simulink model "DSM6"  (R2020a)
settings: Solver=VariableStepAuto  StartTime=0.0  StopTime=0.3  RelTol=1e-3
settings Model: Creator=86188  LastModifiedBy=bzhan
settings DataIOCC: ReturnWorkspaceOutputs=off
settings DebuggingCC: ArithmeticOperatorsInVariantConditions=warning
settings SFSimCC: SimUseLocalCustomCode=off  CustomCodeUndefinedFunction=UseInterfaceOnly
settings RTWCC: RTWUseLocalCustomCode=off

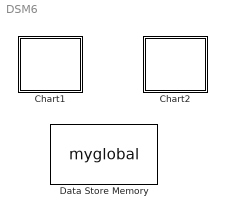
== system DSM6 ==
  Chart1 : Stateflow chart  TreatAsAtomicUnit=on
  Chart2 : Stateflow chart  TreatAsAtomicUnit=on
  Data Store Memory : DataStoreMemory  DataStoreName=myglobal  ReadBeforeWriteMsg=warning  WriteAfterWriteMsg=warning  WriteAfterReadMsg=warning  InitialValue=[0,0]  ShowAdditionalParam=off  OutDataTypeStr=int32

== stateflow chart DSM6/Chart2 ==
  settings: updateMethod=DISCRETE  sampleTime=0.1
  state A1
    en:f("en_A1");
    myglobal(2)=4;
    du:f("du_A1");
  (default) -> A1
  data: s function_input; myglobal data_store_memory
  function f(s):
    | function f(s)
    |   fprintf(s+" %d %d\n", myglobal(1), myglobal(2));

== stateflow chart DSM6/Chart1 ==
  settings: updateMethod=DISCRETE  sampleTime=0.1
  state A
    en: f("en_A");
    [myglobal(1)]=duA();
  state B
    en:f("en_B");
    myglobal(2)=0;
  (default) -> A
  A -> B : {myglobal(1) = myglobal(1)+1;
      |  y=myglobal(1);}
  B -> A : {myglobal(2)=myglobal(2)-1;
      | y=myglobal(2);}
  data: y1 function_output; s function_input; myglobal data_store_memory; y local int32
  function y1 = duA:
    | function y1 = duA
    |   y1=3;
  function f(s):
    | function f(s)
    |   fprintf(s+" %d %d\n", myglobal(1), myglobal(2));
